simulink subsystem "k64f_hardware_subsystem"  (R2020a)
settings: Solver=VariableStepAuto  StartTime=0.0  StopTime=10.0  RelTol=1e-3
undefined symbols (not defined in the file): A0, A1, A2, A3, A4, D0, D1, D10, D11, D12, D13, D2, D3, D4, D5, D6, D7, D8, D9, PTA0, PTA1, PTA2, PTB10, PTB11, PTB2, PTB23, PTB3, PTB9, PTC11, PTC16, PTC17, PTC2, PTC3, PTC4, PTD0, PTD1, PTD2, PTD3
libraries: frdmk64flib x19
settings Model: Creator=Tim_G  LastModifiedBy=Tim_G

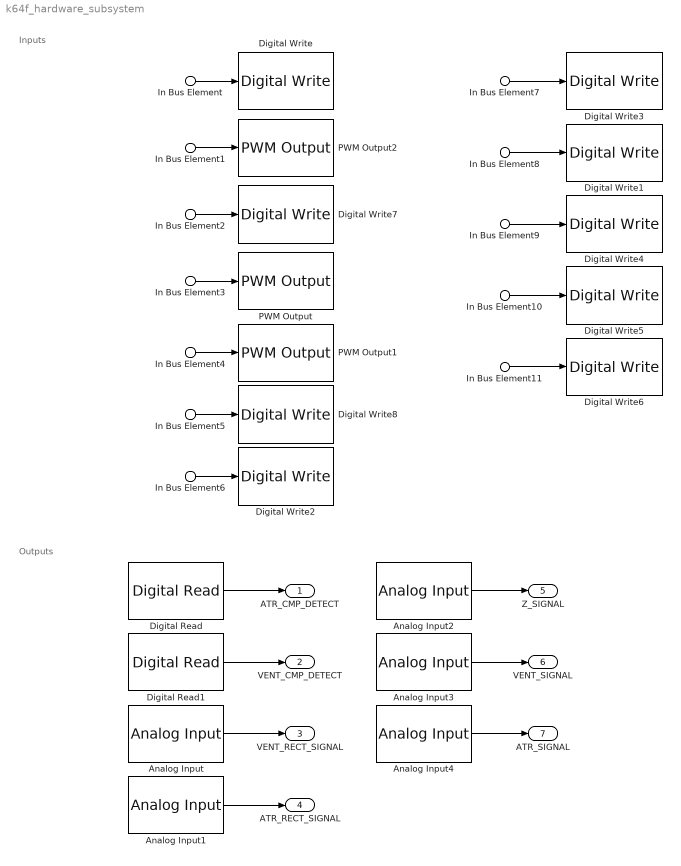
== system k64f_hardware_subsystem ==
  note: Inputs
  note: Outputs
  In Bus Element : Inport  PortName=ControlBus  Element=PACE_CHARGE_CTRL
  In Bus Element1 : Inport  PortName=ControlBus  Element=VENT_CMP_REF_PWM
  In Bus Element2 : Inport  PortName=ControlBus  Element=Z_ATR_CTRL
  In Bus Element3 : Inport  PortName=ControlBus  Element=PACING_REF_PWM
  In Bus Element4 : Inport  PortName=ControlBus  Element=ATR_CMP_REF_PWM
  In Bus Element5 : Inport  PortName=ControlBus  Element=Z_VENT_CTRL
  In Bus Element6 : Inport  PortName=ControlBus  Element=ATR_PACE_CTRL
  In Bus Element7 : Inport  PortName=ControlBus  Element=VENT_PACE_CTRL
  In Bus Element8 : Inport  PortName=ControlBus  Element=PACE_GND_CTRL
  In Bus Element9 : Inport  PortName=ControlBus  Element=ATR_GND_CTRL
  In Bus Element10 : Inport  PortName=ControlBus  Element=VENT_GND_CTRL
  In Bus Element11 : Inport  PortName=ControlBus  Element=FRONTEND_CTRL
  Analog Input : frdmk64flib/Analog Input  Whichpin=PTC11 (A4)  SampleTime=-1
  Analog Input1 : frdmk64flib/Analog Input  Whichpin=PTB11 (A3)  SampleTime=-1
  Analog Input2 : frdmk64flib/Analog Input  Whichpin=PTB10 (A2)  SampleTime=-1
  Analog Input3 : frdmk64flib/Analog Input  Whichpin=PTB3 (A1)  SampleTime=-1
  Analog Input4 : frdmk64flib/Analog Input  Whichpin=PTB2 (A0)  SampleTime=-1
  Digital Read : frdmk64flib/Digital Read  Whichpin=PTC16 (D0)  SampleTime=-1
  Digital Read1 : frdmk64flib/Digital Read  Whichpin=PTC17 (D1)  SampleTime=-1
  Digital Write : frdmk64flib/Digital Write  Whichpin=PTB9 (D2)
  Digital Write1 : frdmk64flib/Digital Write  Whichpin=PTD0 (D10)
  Digital Write2 : frdmk64flib/Digital Write  Whichpin=PTA0 (D8)
  Digital Write3 : frdmk64flib/Digital Write  Whichpin=PTC4 (D9)
  Digital Write4 : frdmk64flib/Digital Write  Whichpin=PTD2 (D11)
  Digital Write5 : frdmk64flib/Digital Write  Whichpin=PTD3 (D12)
  Digital Write6 : frdmk64flib/Digital Write  Whichpin=PTD1 (D13)
  Digital Write7 : frdmk64flib/Digital Write  Whichpin=PTB23 (D4)
  Digital Write8 : frdmk64flib/Digital Write  Whichpin=PTC3 (D7)
  PWM Output : frdmk64flib/PWM Output  Whichpin=PTA2 (D5)  InitialFrequency=2000  InitialDutyCycle=0
  PWM Output1 : frdmk64flib/PWM Output  Whichpin=PTC2 (D6)  InitialFrequency=2000  InitialDutyCycle=0
  PWM Output2 : frdmk64flib/PWM Output  Whichpin=PTA1 (D3)  InitialFrequency=2000  InitialDutyCycle=0
  ATR_CMP_DETECT : Outport
  VENT_CMP_DETECT : Outport  Port=2
  VENT_RECT_SIGNAL : Outport  Port=3
  ATR_RECT_SIGNAL : Outport  Port=4
  Z_SIGNAL : Outport  Port=5
  VENT_SIGNAL : Outport  Port=6
  ATR_SIGNAL : Outport  Port=7
  wires:
  In Bus Element/1 -> Digital Write/1
  In Bus Element1/1 -> PWM Output2/1
  In Bus Element3/1 -> PWM Output/1
  In Bus Element4/1 -> PWM Output1/1
  In Bus Element6/1 -> Digital Write2/1
  In Bus Element7/1 -> Digital Write3/1
  In Bus Element8/1 -> Digital Write1/1
  In Bus Element9/1 -> Digital Write4/1
  In Bus Element10/1 -> Digital Write5/1
  In Bus Element11/1 -> Digital Write6/1
  Digital Read/1 -> ATR_CMP_DETECT/1
  Digital Read1/1 -> VENT_CMP_DETECT/1
  Analog Input/1 -> VENT_RECT_SIGNAL/1
  Analog Input1/1 -> ATR_RECT_SIGNAL/1
  In Bus Element2/1 -> Digital Write7/1
  In Bus Element5/1 -> Digital Write8/1
  Analog Input2/1 -> Z_SIGNAL/1
  Analog Input3/1 -> VENT_SIGNAL/1
  Analog Input4/1 -> ATR_SIGNAL/1
